simulink model "nms_3Dmodel_mld"  (R2019a)
settings: Solver=ode15s  StartTime=0.0  StopTime=7  FixedStep=1e-3  RelTol=1e-3  AbsTol=1e-4  EnableMultiTasking=on
InitFcn:
  | runScripts;
undefined symbols (not defined in the file or in its folder): ankle_height, c, c_jointstop, CtrlPar_FP, CtrlPar_FP_R, CtrlPar_LL, CtrlPar_St, CtrlPar_St_R, CtrlPar_Sw, CtrlPar_Sw_R, CtrlPar_theta0, CtrlPar_Tr, CtrlPar_Tr_R, D12_F, D12_S, D12_T, D12z_T, D13_F, D1G_F, D1G_HAT, D1G_S, D1G_T, D1Gy_F, d_fBall, d_fHeel, DeltaThRef, dt, eref, FmaxBFSH, FmaxGAS, FmaxGLU, FmaxHAB, FmaxHAD, FmaxHAM, FmaxHFL, FmaxRF, FmaxSOL, FmaxTA, FmaxVAS, In_F, In_HAT, In_S, In_T, init_a_tgt, init_a_tgtR, Inx_F, Inx_HAT, Inx_S, Inx_T, Iny_F, Iny_HAT, Iny_S, Iny_T, K, k_gn, k_gt, k_pressure, leg_l, LongDelay, LongLoopDelay ... (+139)
libraries: mblibv1 x89, simulink x44, simulink_extras x38
(part 1 of 13)
settings Model: Creator=hgeyer  LastModifiedBy=Jesper
settings SolverCC: AutoScaleAbsTol=off  ZeroCrossAlgorithm=Adaptive
settings DataIOCC: SaveFormat=StructureWithTime  SignalLoggingSaveFormat=ModelDataLogs  SaveState=on
settings OptimizationCC: BooleanDataType=off  ExpressionDepthLimit=2147483647  InitFltsAndDblsToZero=on  LifeSpan=inf
settings DebuggingCC: SaveWithParameterizedLinksMsg=none  UnderspecifiedInitializationDetection=Classic  MergeDetectMultiDrivingBlocksExec=none  SignalResolutionControl=TryResolveAllWithWarning  MaxConsecutiveZCsMsg=warning  SolverPrmCheckMsg=warning  MultiTaskDSMMsg=warning  MultiTaskCondExecSysMsg=none  FcnCallInpInsideContextMsg=warning  UnconnectedLineMsg=none  StateNameClashWarn=warning  SFUnexpectedBacktrackingDiag=warning  SFNoUnconditionalDefaultTransitionDiag=warning  SFExecutionAtInitializationDiag=none  ArithmeticOperatorsInVariantConditions=warning
settings HardwareCC: ProdBitPerPointer=32  ProdBitPerSizeT=32  ProdBitPerPtrDiffT=32  ProdLargestAtomicFloat=None  ProdIntDivRoundTo=Undefined  ProdEndianess=Unspecified  ProdWordSize=32  ProdHWDeviceType=32-bit Generic
settings ModelReferenceCC: PropagateSignalLabelsOutOfModel=off
settings SFSimCC: SimUseLocalCustomCode=off
settings RTWCC: RTWUseLocalCustomCode=off
settings CodeAppCC: StateflowObjectComments=on
settings GRTTargetCC: TargetFcnLib=ansi_tfl_tmw.mat  TargetLangStandard=C89/C90 (ANSI)  GeneratePreprocessorConditionals=Disable all  CombineOutputUpdateFcns=off  GRTInterface=on
settings ConfigComp: CovMetricSettings=dw  CovHtmlReporting=on  CovSaveCumulativeToWorkspaceVar=on  CovSaveSingleToWorkspaceVar=on  CovExternalEMLEnable=off
settings SimscapeCC: SimscapeNormalizeSystem=off
settings SimMechanicsCC: VisOnUpdateDiagram=on  VisDuringSimulation=on  VisSampleTime=0.01  HighlightModel=off  AutoFitVis=GROWTOFIT  LastVizWinPosition=[126 112 1245 592]  CamPosition=[10.9406;3.67889;8.45305;]  CamTarget=[0.97968;0.591012;-0.112655;]  CamUpVector=[-0.166765;0.973419;-0.156985;]  CamHeight=3.15748  VisBackgroundColor=[0.9;0.9;0.95;]  DefaultBodyColor=[1;0;0;]
settings ConfigurationSet: Description=SimMechanics 2G

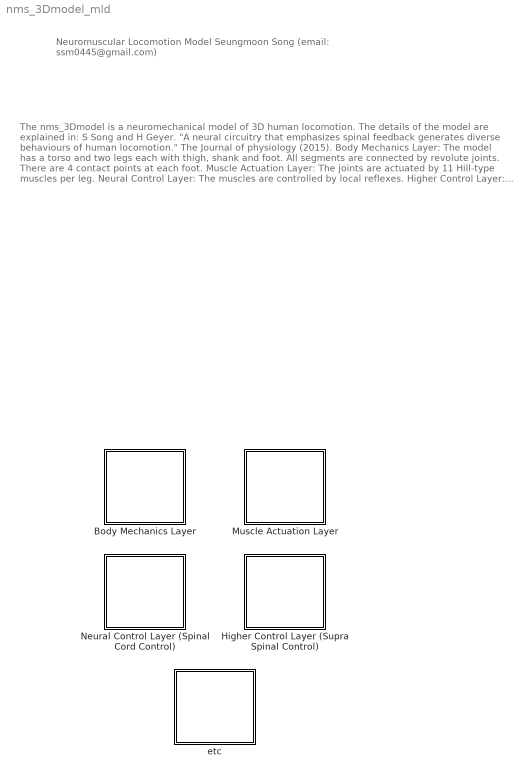
== system nms_3Dmodel_mld ==
  note: Neuromuscular Locomotion Model
      | Seungmoon Song
      | (email: ssm0445@gmail.com)
  note: The nms_3Dmodel is a neuromechanical model of 3D human locomotion.
      | The details of the model are explained in:
      | S Song and H Geyer. "A neural circuitry that emphasizes spinal feedback
      | generates diverse behaviours of human locomotion." The Journal of physiology (2015).
      |
      | Body Mechanics Layer:
      | The model has a torso and two legs each with thigh, shank and foot.
      | All segments are connected by revolute joints.
      | There are 4 contact points at each foot.
      |
      | Muscle Actuation Layer:
      | The joints are actuated by 11 Hill-type muscles per leg.
      |
      | Neural Control Layer:
      | The muscles are controlled by local reflexes.
      |
      | Higher Control Layer:
      | The reflex pathways are modulated by the higher layer control.
  Body Mechanics Layer : Subsystem
  Higher Control Layer (Supra Spinal Control) : Subsystem
  Muscle Actuation Layer : Subsystem
  Neural Control Layer (Spinal Cord Control) : Subsystem
  etc : Subsystem
